simulink model "Electrical787"  (R2013a)
settings: Solver=ode45  StartTime=0.0  StopTime=MSSN.gen.time(end)  RelTol=1e-3
InitFcn:
  | load('SampleOutput.mat')
  | 
  | load('SampleFuelBurn.mat')
undefined symbols (not defined in the file): ailerons, B_737, elevator, FuelBurn, landing_gear, rudder, thrust_rev
libraries: PowerFlowLib x95, simulink x17
(part 17 of 17)

== system Electrical787/ELECTRICAL SYS /Engine Outputs ==
  Left_Wing_Toqrue_Nm : Inport
  Rght_Wing_Torque_Nm : Inport  Port=2
  APU_Torque_Nm : Inport  Port=3
  Bus Creator : BusCreator  Inputs=3
  Electrical : Outport
  wires:
  Rght_Wing_Torque_Nm/1 -> Bus Creator/2  "Right Wing Torq (Nm)"
  APU_Torque_Nm/1 -> Bus Creator/3  "APU Torq (Nm)"
  Left_Wing_Toqrue_Nm/1 -> Bus Creator/1  "Left Wing Torq (Nm)"
  Bus Creator/1 -> Electrical/1

== system Electrical787/ELECTRICAL SYS /Generation Unit P.M. ==
  engine speed : Inport
  idq0 : Inport  Port=2
  Temperature : Inport  Port=3
  Bus Creator : BusCreator  Inputs=3
  Bus Creator1 : BusCreator  Inputs=3
  Coeff of Resistance : Gain  Gain=3.85e-3
  Demux : Demux  Outputs=3
  Gain : Gain  Gain=200*2/3
  Gain1 : Gain  Gain=200
  Generator : Subsystem
      mask Display:
      | p = 0:0.1:(2*pi+0.1);
      | plot(sin(p), cos(p));
      | p1 = (-pi/8-0.1-0.2):0.1:(pi/8+0.1-0.2);
      | plot(0.8*sin(p1), 0.8*cos(p1), 0.8*sin(p1+pi), 0.8*cos(p1+pi));
      | p2 = sin((-pi/8-0.1-0.2+pi/8+0.1-0.2)/2);
      | p3 = sin((-pi/8-0.1-0.2+pi/8+0.1-0.2)/2+pi);
      | p4 = cos((-pi/8-0.1-0.2+pi/8+0.1-0.2)/2);
      | p5 = cos((-pi/8-0.1-0.2+pi/8+0.1-0.2)/2+pi);
      | plot(0.8*[p2, p3], 0.8*[p4, p5]);
      | port_label('output', 1, 'Vdq0');
      | port_label('output', 2, 'Te');
      | port_label('output', 3, 'Vfd');
      | port_label('output', 4, 'Ploss');
      | port_label('input', 1, 'idq0');
      | port_label('input', 2, 'w');
      | port_label('input', 3, 'ifd');
  Initial Temperature : Constant  Value=25
  Memory : Memory
  Permanent Magnet Synchronous Generator1 : PowerFlowLib/Energy & Power Systems/Electrical/Machines/Permanent Magnet Synchronous Generator1
  RPM_to_radps : Gain  Gain=pi/30
  Scope2 : Scope
      settings: TimeRange=100  YMin=0  YMax=5500  SaveName=ScopeData4
  Sum : Sum  Inputs=++|
  Sum1 : Sum
  Sum5 : Sum  Inputs=|+-
  Sum6 : Sum  Inputs=|++
  control1 : Constant
  data_sink : PowerFlowLib/Support Functions//Tools/data_sink
  one : Constant
  three-phase active rectifier Voltage Mode : PowerFlowLib/Energy & Power Systems/Electrical/Rectifiers/three-phase  active rectifier Voltage Mode  L=1  C=1e-4
  vdq0 : Outport
  engine torque : Outport  Port=2
  Ploss : Outport  Port=3
  wires:
  [R_temp_delta] -> Generator/4(Temp)
  Sum6/1 -> [R_temp_delta]
  one/1 -> Sum6/2
  Coeff of Resistance/1 -> Sum6/1
  Sum5/1 -> Coeff of Resistance/1
  Initial Temperature/1 -> Sum5/2
  Temperature/1 -> Sum5/1
  engine speed/1 -> RPM_to_radps/1
  Bus Creator1/1 -> Bus Creator/1  "vdq0 (V)"
  Demux/3 -> Bus Creator1/3  "v0"
  Demux/2 -> Bus Creator1/2  "vq"
  Demux/1 -> Bus Creator1/1  "vd"
  Bus Creator/1 -> data_sink/1
  Sum/1 -> engine torque/1
  RPM_to_radps/1 -> Scope2/1, Permanent Magnet Synchronous Generator1/2, Generator/2(w)
  Permanent Magnet Synchronous Generator1/1 -> three-phase active rectifier Voltage Mode/1
  control1/1 -> three-phase active rectifier Voltage Mode/2
  Generator/3(vfd') -> Gain1/1
  Gain1/1 -> three-phase active rectifier Voltage Mode/3
  Gain/1 -> Generator/3(ifd'), Bus Creator/3  "Excit current (A)"
  three-phase active rectifier Voltage Mode/1 -> Gain/1
  three-phase active rectifier Voltage Mode/2 -> Memory/1
  Permanent Magnet Synchronous Generator1/2 -> Sum/1
  Generator/2(Te) -> Sum/2
  idq0/1 -> Generator/1(idq0)
  Generator/1(vdq0) -> Demux/1, vdq0/1  "Vdq0 (V)"
  Permanent Magnet Synchronous Generator1/3 -> Sum1/1
  Generator/4(Ploss) -> Sum1/2
  Sum1/1 -> Bus Creator/2, Ploss/1  "Ploss (W)"
  Memory/1 -> Permanent Magnet Synchronous Generator1/1

== system Electrical787/ELECTRICAL SYS /Generation Unit P.M.1 ==
  engine speed : Inport
  idq0 : Inport  Port=2
  Temperature : Inport  Port=3
  Bus Creator : BusCreator  Inputs=3
  Bus Creator1 : BusCreator  Inputs=3
  Coeff of Resistance : Gain  Gain=3.85e-3
  Demux : Demux  Outputs=3
  Gain : Gain  Gain=200*2/3
  Gain1 : Gain  Gain=200
  Generator : Subsystem
      mask Display:
      | p = 0:0.1:(2*pi+0.1);
      | plot(sin(p), cos(p));
      | p1 = (-pi/8-0.1-0.2):0.1:(pi/8+0.1-0.2);
      | plot(0.8*sin(p1), 0.8*cos(p1), 0.8*sin(p1+pi), 0.8*cos(p1+pi));
      | p2 = sin((-pi/8-0.1-0.2+pi/8+0.1-0.2)/2);
      | p3 = sin((-pi/8-0.1-0.2+pi/8+0.1-0.2)/2+pi);
      | p4 = cos((-pi/8-0.1-0.2+pi/8+0.1-0.2)/2);
      | p5 = cos((-pi/8-0.1-0.2+pi/8+0.1-0.2)/2+pi);
      | plot(0.8*[p2, p3], 0.8*[p4, p5]);
      | port_label('output', 1, 'Vdq0');
      | port_label('output', 2, 'Te');
      | port_label('output', 3, 'Vfd');
      | port_label('output', 4, 'Ploss');
      | port_label('input', 1, 'idq0');
      | port_label('input', 2, 'w');
      | port_label('input', 3, 'ifd');
  Initial Temperature : Constant  Value=25
  Memory : Memory
  Permanent Magnet Synchronous Generator1 : PowerFlowLib/Energy & Power Systems/Electrical/Machines/Permanent Magnet Synchronous Generator1
  RPM_to_radps : Gain  Gain=pi/30
  Scope2 : Scope
      settings: TimeRange=100  YMin=0  YMax=5500  SaveName=ScopeData4
  Sum : Sum  Inputs=++|
  Sum1 : Sum
  Sum5 : Sum  Inputs=|+-
  Sum6 : Sum  Inputs=|++
  control1 : Constant
  data_sink : PowerFlowLib/Support Functions//Tools/data_sink
  one : Constant
  three-phase active rectifier Voltage Mode : PowerFlowLib/Energy & Power Systems/Electrical/Rectifiers/three-phase  active rectifier Voltage Mode  L=1  C=1e-4
  vdq0 : Outport
  engine torque : Outport  Port=2
  Ploss : Outport  Port=3
  wires:
  [R_temp_delta] -> Generator/4(Temp)
  Sum6/1 -> [R_temp_delta]
  one/1 -> Sum6/2
  Coeff of Resistance/1 -> Sum6/1
  Sum5/1 -> Coeff of Resistance/1
  Initial Temperature/1 -> Sum5/2
  Temperature/1 -> Sum5/1
  engine speed/1 -> RPM_to_radps/1
  Bus Creator1/1 -> Bus Creator/1  "vdq0 (V)"
  Demux/3 -> Bus Creator1/3  "v0"
  Demux/2 -> Bus Creator1/2  "vq"
  Demux/1 -> Bus Creator1/1  "vd"
  Bus Creator/1 -> data_sink/1
  Sum/1 -> engine torque/1
  RPM_to_radps/1 -> Scope2/1, Permanent Magnet Synchronous Generator1/2, Generator/2(w)
  Permanent Magnet Synchronous Generator1/1 -> three-phase active rectifier Voltage Mode/1
  control1/1 -> three-phase active rectifier Voltage Mode/2
  Generator/3(vfd') -> Gain1/1
  Gain1/1 -> three-phase active rectifier Voltage Mode/3
  Gain/1 -> Generator/3(ifd'), Bus Creator/3  "Excit current (A)"
  three-phase active rectifier Voltage Mode/1 -> Gain/1
  three-phase active rectifier Voltage Mode/2 -> Memory/1
  Permanent Magnet Synchronous Generator1/2 -> Sum/1
  Generator/2(Te) -> Sum/2
  idq0/1 -> Generator/1(idq0)
  Generator/1(vdq0) -> Demux/1, vdq0/1  "Vdq0 (V)"
  Permanent Magnet Synchronous Generator1/3 -> Sum1/1
  Generator/4(Ploss) -> Sum1/2
  Sum1/1 -> Bus Creator/2, Ploss/1  "Ploss (W)"
  Memory/1 -> Permanent Magnet Synchronous Generator1/1

== system Electrical787/ELECTRICAL SYS /Loads ==
  Constant{,1..3} (4 alike) : Constant  Value=[150 0 0]
  ElectricalSource1 : PowerFlowLib/Support Functions//Tools/ElectricalSource  Tag=Flow  Description=TwoPhase  load_loc=Cockpit  ACDC_load=DC
      link override From1: GotoTag=RightWing_ElecAC_9219
      link override From2: GotoTag=RightWing_ElecAC_5921
  ElectricalSource4 : PowerFlowLib/Support Functions//Tools/ElectricalSource  Tag=Flow  Description=TwoPhase  load_loc=RightWing  ACDC_load=AC
      link override From1: GotoTag=RightWing_ElecAC_9219
      link override From2: GotoTag=RightWing_ElecAC_5921
  ElectricalSource5 : PowerFlowLib/Support Functions//Tools/ElectricalSource  Tag=Flow  Description=TwoPhase  load_loc=RightWing  ACDC_load=AC
      link override From1: GotoTag=RightWing_ElecAC_9219
      link override From2: GotoTag=RightWing_ElecAC_5921
  ElectricalSource6 : PowerFlowLib/Support Functions//Tools/ElectricalSource  Tag=Flow  Description=TwoPhase  load_loc=Cabin  ACDC_load=DC
      link override From1: GotoTag=RightWing_ElecAC_9219
      link override From2: GotoTag=RightWing_ElecAC_5921
  Reactive Power : Gain  Gain=[0 1 0]
  Reactive Power1 : Gain  Gain=[0 1 0]
  "Real Power " : Gain  Gain=[0 1]
  "Real Power  " : Gain  Gain=[1 0 0]
  Real Power  1 : Gain  Gain=[1 0 0]
  Real Power 1 : Gain  Gain=[0 1]
  Sum : Sum  Inputs=|++
  Sum of Elements{,1..3} (4 alike) : Sum  Inputs=+
  Sum1 : Sum  Inputs=|++
  230 Vac Loads : Outport
  115 Vac Loads : Outport  Port=2
  270 Vdc Loads : Outport  Port=3
  28 Vdc Loads : Outport  Port=4
  wires:
  "Real Power  "/1 -> Sum/1
  Reactive Power/1 -> Sum/2
  Sum of Elements/1 -> "Real Power  "/1
  Sum of Elements1/1 -> Reactive Power/1
  Real Power  1/1 -> Sum1/1
  Reactive Power1/1 -> Sum1/2
  Sum of Elements2/1 -> Real Power  1/1
  Sum of Elements3/1 -> Reactive Power1/1
  ElectricalSource6/1 -> "Real Power "/1
  ElectricalSource4/2 -> Sum of Elements3/1
  ElectricalSource5/1 -> Sum of Elements/1
  ElectricalSource5/2 -> Sum of Elements1/1
  ElectricalSource4/1 -> Sum of Elements2/1
  ElectricalSource1/1 -> Real Power 1/1
  Constant/1 -> 230 Vac Loads/1
  Constant1/1 -> 115 Vac Loads/1
  Constant2/1 -> 270 Vdc Loads/1
  Constant3/1 -> 28 Vdc Loads/1

== system Electrical787/ELECTRICAL SYS /Thermal Interface ==
  Left_Wing_SCVGU_Ploss_W : Inport
  Right_Wing_SCVGU_Ploss_W : Inport  Port=2
  APU_Ploss_W : Inport  Port=3
  Inverter_Ploss_W : Inport  Port=4
  Battery1_Ploss_W : Inport  Port=5
  Battery2_Ploss_W : Inport  Port=6
  Backup_Battery_Ploss_W : Inport  Port=7
  Loadloss_W : Inport  Port=8
  Mux : Mux
  Sum : Sum
  Terminator{,1..3} (4 alike) : Terminator
  ThermalSink : PowerFlowLib/Support Functions//Tools/ThermalSink  Tag=Flow  Description=TwoPhase  load_loc=Cabin  units=Watts  unq_id=8332
  To Workspace : ToWorkspace  VariableName=Tot_Gen_Loss_W  SampleTime=10  SaveFormat=Structure With Time
  wires:
  Right_Wing_SCVGU_Ploss_W/1 -> Sum/2, Terminator1/1
  APU_Ploss_W/1 -> Terminator2/1
  Mux/1 -> ThermalSink/1
  Inverter_Ploss_W/1 -> Mux/1
  Battery1_Ploss_W/1 -> Mux/2
  Battery2_Ploss_W/1 -> Mux/3
  Backup_Battery_Ploss_W/1 -> Mux/4
  Loadloss_W/1 -> Terminator3/1
  Left_Wing_SCVGU_Ploss_W/1 -> Sum/1, Terminator/1
  Sum/1 -> To Workspace/1

== system Electrical787/Engine #1/Unit Conversion  ==
  Signal_in : Inport
  conv_fcn : Fcn  Expr=u(1)/745.69987
  Converted Signal Out : Outport
  wires:
  Signal_in/1 -> conv_fcn/1
  conv_fcn/1 -> Converted Signal Out/1

== system Electrical787/Engine #1/Unit Conversion 1 ==
  Signal_in : Inport
  conv_fcn : Fcn  Expr=u(1)/1.8
  Converted Signal Out : Outport
  wires:
  conv_fcn/1 -> Converted Signal Out/1
  Signal_in/1 -> conv_fcn/1

== system Electrical787/Engine #1/Unit Conversion 2 ==
  Signal_in : Inport
  conv_fcn : Fcn  Expr=u(1)/.45359237
  Converted Signal Out : Outport
  wires:
  conv_fcn/1 -> Converted Signal Out/1
  Signal_in/1 -> conv_fcn/1

== system Electrical787/Engine #1/Unit Conversion 3 ==
  Signal_in : Inport
  conv_fcn : Fcn  Expr=u(1)/.45359237
  Converted Signal Out : Outport
  wires:
  conv_fcn/1 -> Converted Signal Out/1
  Signal_in/1 -> conv_fcn/1

== system Electrical787/Engine #1/Unit Conversion 4 ==
  Signal_in : Inport
  conv_fcn : Fcn  Expr=u(1)/(1.450377e-1)
  Converted Signal Out : Outport
  wires:
  Signal_in/1 -> conv_fcn/1
  conv_fcn/1 -> Converted Signal Out/1

== system Electrical787/Engine #1/Unit Conversion 5 ==
  Signal_in : Inport
  conv_fcn : Fcn  Expr=u(1)*.45359237
  Converted Signal Out : Outport
  wires:
  Signal_in/1 -> conv_fcn/1
  conv_fcn/1 -> Converted Signal Out/1

== system Electrical787/Engine #2/Unit Conversion  ==
  Signal_in : Inport
  conv_fcn : Fcn  Expr=u(1)/745.69987
  Converted Signal Out : Outport
  wires:
  conv_fcn/1 -> Converted Signal Out/1
  Signal_in/1 -> conv_fcn/1

== system Electrical787/Engine #2/Unit Conversion 1 ==
  Signal_in : Inport
  conv_fcn : Fcn  Expr=u(1)/1.8
  Converted Signal Out : Outport
  wires:
  Signal_in/1 -> conv_fcn/1
  conv_fcn/1 -> Converted Signal Out/1

== system Electrical787/Engine #2/Unit Conversion 2 ==
  Signal_in : Inport
  conv_fcn : Fcn  Expr=u(1)/.45359237
  Converted Signal Out : Outport
  wires:
  Signal_in/1 -> conv_fcn/1
  conv_fcn/1 -> Converted Signal Out/1

== system Electrical787/Engine #2/Unit Conversion 3 ==
  Signal_in : Inport
  conv_fcn : Fcn  Expr=u(1)/.45359237
  Converted Signal Out : Outport
  wires:
  Signal_in/1 -> conv_fcn/1
  conv_fcn/1 -> Converted Signal Out/1

== system Electrical787/Engine #2/Unit Conversion 4 ==
  Signal_in : Inport
  conv_fcn : Fcn  Expr=u(1)/(1.450377e-1)
  Converted Signal Out : Outport
  wires:
  conv_fcn/1 -> Converted Signal Out/1
  Signal_in/1 -> conv_fcn/1

== system Electrical787/Engine #2/Unit Conversion 5 ==
  Signal_in : Inport
  conv_fcn : Fcn  Expr=u(1)*.45359237
  Converted Signal Out : Outport
  wires:
  conv_fcn/1 -> Converted Signal Out/1
  Signal_in/1 -> conv_fcn/1

== system Electrical787/ECS & FOS /Fuel Tanks//Pumps/FlowGenerator1 ==
  Bias : Bias  Bias=273.15
  Bus Creator1 : BusCreator
  Constant3 : Constant  Value=flowenthalpy
  Constant5 : Constant  Value=flowrate
  Constant6 : Constant  Value=flowtemp
  Constant7 : Constant  Value=flowpres
  FlowOut : Outport  Tag=Flow Out
  wires:
  Bias/1 -> Bus Creator1/2  "temp_K"
  Constant5/1 -> Bus Creator1/1  "mdot_kgps"
  Constant3/1 -> Bus Creator1/4  "H_kJpkg"
  Constant7/1 -> Bus Creator1/3  "pres_kPa"
  Constant6/1 -> Bias/1  "temp_C"
  Bus Creator1/1 -> FlowOut/1  "Outlet"

== system Electrical787/ECS & FOS /Fuel Tanks//Pumps/Fuel Control Left Wing ==
  FuelNeed : Inport
  FuelFromPump : Inport  Port=2
  Bus Creator : BusCreator  Inputs=3
  Bus Creator1 : BusCreator  Inputs=3
  Bus Selector : BusSelector  OutputSignals=mdot_kgps,temp_K,pres_kPa
  Gain : Gain
  Gain1 : Gain
  Saturation : Saturate  UpperLimit=inf  LowerLimit=0
  Sum : Sum  Inputs=|+-
  Switch : Switch  Criteria=u2 > Threshold
  Fuel2Engine : Outport
  Fuel2Tank : Outport  Port=2
  wires:
  Gain1/1 -> Bus Creator1/2  "temp_K"
  Gain/1 -> Bus Creator1/3  "pres_kPa"
  Bus Creator1/1 -> Fuel2Engine/1
  Bus Selector/3 -> Gain/1, Bus Creator/3  "<pres_kPa>"
  Switch/1 -> Bus Creator1/1  "mdot_kgps"
  Saturation/1 -> Bus Creator/1  "mdot_kgps"
  Bus Selector/2 -> Gain1/1, Bus Creator/2  "<temp_K>"
  Bus Creator/1 -> Fuel2Tank/1
  Sum/1 -> Switch/2, Saturation/1
  FuelNeed/1 -> Switch/1, Sum/2
  Bus Selector/1 -> Switch/3, Sum/1  "<mdot_kgps>"
  FuelFromPump/1 -> Bus Selector/1

== system Electrical787/ECS & FOS /Fuel Tanks//Pumps/Fuel Control Right Wing  ==
  FuelNeed : Inport
  FuelFromPump : Inport  Port=2
  Bus Creator : BusCreator  Inputs=3
  Bus Creator1 : BusCreator  Inputs=3
  Bus Selector : BusSelector  OutputSignals=mdot_kgps,temp_K,pres_kPa
  Gain : Gain
  Gain1 : Gain
  Saturation : Saturate  UpperLimit=inf  LowerLimit=0
  Sum : Sum  Inputs=|+-
  Switch : Switch  Criteria=u2 > Threshold
  Fuel2Engine : Outport
  Fuel2Tank : Outport  Port=2
  wires:
  FuelFromPump/1 -> Bus Selector/1
  Bus Selector/1 -> Sum/1, Switch/3  "<mdot_kgps>"
  FuelNeed/1 -> Sum/2, Switch/1
  Sum/1 -> Saturation/1, Switch/2
  Bus Creator/1 -> Fuel2Tank/1
  Bus Selector/2 -> Bus Creator/2, Gain1/1  "<temp_K>"
  Saturation/1 -> Bus Creator/1  "mdot_kgps"
  Switch/1 -> Bus Creator1/1  "mdot_kgps"
  Bus Selector/3 -> Bus Creator/3, Gain/1  "<pres_kPa>"
  Bus Creator1/1 -> Fuel2Engine/1
  Gain/1 -> Bus Creator1/3  "pres_kPa"
  Gain1/1 -> Bus Creator1/2  "temp_K"

== system Electrical787/ECS & FOS /Fuel Tanks//Pumps/Fuel Switch On//Off ==
  Right Wing Tank : Inport
  Center Tank : Inport  Port=2
  Left Wing Tank : Inport  Port=3
  Operating RPM : Constant  Value=6000
  Operating RPM1 : Constant  Value=6000
  Operating RPM2 : Constant  Value=6000
  Right Wing Fuel Pumps On/Off : Switch  Criteria=u2 ~= 0
  Right Wing Fuel Pumps On/Off1 : Switch  Criteria=u2 ~= 0
  Right Wing Fuel Pumps On/Off2 : Switch  Criteria=u2 ~= 0
  shut off : Constant  Value=0
  shut off1 : Constant  Value=0
  shut off2 : Constant  Value=0
  Right Wing RPM : Outport
  Left Wing RPM : Outport  Port=2
  Center RPM : Outport  Port=3
  wires:
  Operating RPM/1 -> Right Wing Fuel Pumps On/Off/1
  shut off/1 -> Right Wing Fuel Pumps On/Off/3
  Right Wing Tank/1 -> Right Wing Fuel Pumps On/Off/2
  Operating RPM1/1 -> Right Wing Fuel Pumps On/Off1/1
  shut off1/1 -> Right Wing Fuel Pumps On/Off1/3
  Center Tank/1 -> Right Wing Fuel Pumps On/Off1/2
  Operating RPM2/1 -> Right Wing Fuel Pumps On/Off2/1
  shut off2/1 -> Right Wing Fuel Pumps On/Off2/3
  Left Wing Tank/1 -> Right Wing Fuel Pumps On/Off2/2
  Right Wing Fuel Pumps On/Off/1 -> Right Wing RPM/1
  Right Wing Fuel Pumps On/Off1/1 -> Center RPM/1
  Right Wing Fuel Pumps On/Off2/1 -> Left Wing RPM/1

== system Electrical787/ECS & FOS /Fuel Tanks//Pumps/Pump Split ==
  Flow In : Inport
  Bus Creator : BusCreator  Inputs=3
  Bus Selector14 : BusSelector  OutputSignals=temp_K,mdot_kgps,pres_kPa
  Gain : Gain  Gain=0.5
  Flow Out : Outport
  wires:
  Bus Selector14/3 -> Bus Creator/3  "<pres_kPa>"
  Gain/1 -> Bus Creator/2  "mdot_kgps"
  Bus Selector14/1 -> Bus Creator/1  "<temp_K>"
  Bus Creator/1 -> Flow Out/1
  Bus Selector14/2 -> Gain/1  "<mdot_kgps>"
  Flow In/1 -> Bus Selector14/1

== system Electrical787/ECS & FOS /Fuel Tanks//Pumps/Pump Split1 ==
  Flow In : Inport
  Bus Creator : BusCreator  Inputs=3
  Bus Selector14 : BusSelector  OutputSignals=temp_K,mdot_kgps,pres_kPa
  Gain : Gain  Gain=0.5
  Flow Out : Outport
  wires:
  Flow In/1 -> Bus Selector14/1
  Bus Selector14/2 -> Gain/1  "<mdot_kgps>"
  Bus Creator/1 -> Flow Out/1
  Bus Selector14/1 -> Bus Creator/1  "<temp_K>"
  Gain/1 -> Bus Creator/2  "mdot_kgps"
  Bus Selector14/3 -> Bus Creator/3  "<pres_kPa>"

== system Electrical787/ECS & FOS /Fuel Tanks//Pumps/Pump Split2 ==
  Flow In : Inport
  Bus Creator : BusCreator  Inputs=3
  Bus Selector14 : BusSelector  OutputSignals=temp_K,mdot_kgps,pres_kPa
  Gain : Gain  Gain=0.5
  Flow Out : Outport
  wires:
  Bus Selector14/3 -> Bus Creator/3  "<pres_kPa>"
  Gain/1 -> Bus Creator/2  "mdot_kgps"
  Bus Selector14/1 -> Bus Creator/1  "<temp_K>"
  Bus Creator/1 -> Flow Out/1
  Bus Selector14/2 -> Gain/1  "<mdot_kgps>"
  Flow In/1 -> Bus Selector14/1

== system Electrical787/ECS & FOS /Left PACK/Distribution of bleed air ==
  Bleed to Valve : Inport
  Bleed to ACM : Inport  Port=2
  bleed_temp : Inport  Port=3
  bleed_pres : Inport  Port=4
  Bus Creator1 : BusCreator  Inputs=3
  Bus Creator2 : BusCreator  Inputs=3
  Scope : Scope  NumInputPorts=4
      settings: YMin=0~386.7~110~0.2  YMax=0.055~387.8~160~0.85  SaveName=ScopeData42  SampleInput=on  SampleTime=1
  Flow to Mix Junc. : Outport
  Flow to HX : Outport  Port=2
  wires:
  Bleed to ACM/1 -> Bus Creator2/1, Scope/4  "mdot_kgps"
  bleed_temp/1 -> Bus Creator2/2, Bus Creator1/2, Scope/2
  bleed_pres/1 -> Bus Creator2/3, Bus Creator1/3, Scope/3
  Bleed to Valve/1 -> Bus Creator1/1, Scope/1  "mdot_kgps"
  Bus Creator1/1 -> Flow to Mix Junc./1
  Bus Creator2/1 -> Flow to HX/1

== system Electrical787/ECS & FOS /Left PACK/Ram air inlet ==
  Temp_amb : Inport
  Temp_comp : Inport  Port=2
  2 : Constant  Value=T_35
  Bus Creator : BusCreator  Inputs=3
  Bus Selector4 : BusSelector  OutputSignals=temp_K
  Constant1 : Constant  Value=22.5
  Gain : Gain  Gain=0.95
  Gain1 : Gain
  Memory : Memory  X0=ram_air
  Subtract : Sum  Inputs=+-
  Switch : Switch  Criteria=u2 ~= 0  Threshold=30
  Flow Out : Outport
  wires:
  Temp_comp/1 -> Bus Selector4/1
  Bus Selector4/1 -> Subtract/1  "<temp_K>"
  2/1 -> Subtract/2
  Subtract/1 -> Switch/2
  Gain/1 -> Switch/3
  Switch/1 -> Memory/1
  Temp_amb/1 -> Bus Creator/1  "temp_K"
  Constant1/1 -> Bus Creator/2  "pres_kPa"
  Bus Creator/1 -> Flow Out/1
  Memory/1 -> Bus Creator/3, Gain1/1, Gain/1  "mdot_kgps"
  Gain1/1 -> Switch/1

== system Electrical787/ECS & FOS /Left PACK/Subsystem1 ==
  Bypass Ratio : Inport
  Air from PHX : Inport  Port=2
  Bus Creator : BusCreator  Inputs=3
  Bus Creator1 : BusCreator  Inputs=3
  Bus Selector : BusSelector  OutputSignals=mdot_kgps,temp_K,pres_kPa
  Fcn1 : Fcn  Expr=1-u(1)
  Gain : Gain
  Gain1 : Gain
  Gain2 : Gain
  Product : Product  RndMeth=Zero
  Product1 : Product  RndMeth=Zero
  Saturation : Saturate  UpperLimit=inf  LowerLimit=eps
  Air to Mix Junc : Outport
  Air to Comp : Outport  Port=2
  wires:
  Gain1/1 -> Bus Creator1/2  "temp_K"
  Gain/1 -> Bus Creator1/3  "pres_kPa"
  Bus Creator1/1 -> Air to Mix Junc/1
  Bus Selector/3 -> Gain/1, Gain2/1  "<pres_kPa>"
  Product1/1 -> Bus Creator1/1  "mdot_kgps"
  Saturation/1 -> Bus Creator/1  "mdot_kgps"
  Bus Selector/2 -> Gain1/1, Bus Creator/2  "<temp_K>"
  Bus Creator/1 -> Air to Comp/1
  Bus Selector/1 -> Product/2, Product1/1  "<mdot_kgps>"
  Air from PHX/1 -> Bus Selector/1
  Product/1 -> Saturation/1
  Bypass Ratio/1 -> Fcn1/1, Product1/2
  Fcn1/1 -> Product/1
  Gain2/1 -> Bus Creator/3  "pres_kPa"

== system Electrical787/ECS & FOS /Left PACK/User-set_ supply_pressure ==
  Flow In : Inport
  Cabin Pres. : Inport  Port=2
  Bus Creator4 : BusCreator  Inputs=3
  Bus Selector3 : BusSelector  OutputSignals=mdot_kgps,temp_K
  Gain1 : Gain  Gain=1.1
  Flow Out : Outport
  wires:
  Bus Selector3/1 -> Bus Creator4/1  "<mdot_kgps>"
  Bus Selector3/2 -> Bus Creator4/2  "<temp_K>"
  Gain1/1 -> Bus Creator4/3  "pres_kPa"
  Flow In/1 -> Bus Selector3/1
  Bus Creator4/1 -> Flow Out/1
  Cabin Pres./1 -> Gain1/1

== system Electrical787/ECS & FOS /Left PACK/Valve1 ==
  Flow In : Inport
  Bus Creator2 : BusCreator  Inputs=3
  Bus Selector2 : BusSelector  OutputSignals=mdot_kgps,pres_kPa,temp_K
  Math Functin : Math  Operator=pow  SaturateOnIntegerOverflow=on
  Product : Product  RndMeth=Zero
  Sum : Sum  Inputs=|-+
  "Value?? -- MAW" : Constant  Value=50
  get u : Gain
  mass_flow_rate1 : Constant  Value=2
  Flow Out : Outport
  wires:
  Bus Creator2/1 -> Flow Out/1
  Flow In/1 -> Bus Selector2/1
  Bus Selector2/1 -> Bus Creator2/1, get u/1  "<mdot_kgps>"
  get u/1 -> Math Functin/1
  mass_flow_rate1/1 -> Math Functin/2
  Math Functin/1 -> Product/2
  Product/1 -> Sum/1
  Bus Selector2/2 -> Sum/2  "<pres_kPa>"
  Sum/1 -> Bus Creator2/2  "pres_kPa"
  Bus Selector2/3 -> Bus Creator2/3  "<temp_K>"
  "Value?? -- MAW"/1 -> Product/1

== system Electrical787/ECS & FOS /Right PACK/Distribution of bleed air ==
  Bleed to Valve : Inport
  Bleed to ACM : Inport  Port=2
  bleed_temp : Inport  Port=3
  bleed_pres : Inport  Port=4
  Bus Creator1 : BusCreator  Inputs=3
  Bus Creator2 : BusCreator  Inputs=3
  Scope : Scope  NumInputPorts=4
      settings: YMin=0~386.7~110~0.2  YMax=0.055~387.8~160~0.85  SaveName=ScopeData42  SampleInput=on  SampleTime=1
  Flow to Mix Junc. : Outport
  Flow to HX : Outport  Port=2
  wires:
  Bus Creator2/1 -> Flow to HX/1
  Bus Creator1/1 -> Flow to Mix Junc./1
  Bleed to Valve/1 -> Scope/1, Bus Creator1/1  "mdot_kgps"
  bleed_pres/1 -> Scope/3, Bus Creator1/3, Bus Creator2/3
  bleed_temp/1 -> Scope/2, Bus Creator1/2, Bus Creator2/2
  Bleed to ACM/1 -> Scope/4, Bus Creator2/1  "mdot_kgps"

== system Electrical787/ECS & FOS /Right PACK/Ram air inlet ==
  Temp_amb : Inport
  Temp_comp : Inport  Port=2
  2 : Constant  Value=T_35
  Bus Creator : BusCreator  Inputs=3
  Bus Selector4 : BusSelector  OutputSignals=temp_K
  Constant1 : Constant  Value=22.5
  Gain : Gain  Gain=0.95
  Gain1 : Gain
  Memory : Memory  X0=ram_air
  Subtract : Sum  Inputs=+-
  Switch : Switch  Criteria=u2 ~= 0  Threshold=30
  Flow Out : Outport
  wires:
  Gain1/1 -> Switch/1
  Memory/1 -> Gain/1, Gain1/1, Bus Creator/3  "mdot_kgps"
  Bus Creator/1 -> Flow Out/1
  Constant1/1 -> Bus Creator/2  "pres_kPa"
  Temp_amb/1 -> Bus Creator/1  "temp_K"
  Switch/1 -> Memory/1
  Gain/1 -> Switch/3
  Subtract/1 -> Switch/2
  2/1 -> Subtract/2
  Bus Selector4/1 -> Subtract/1  "<temp_K>"
  Temp_comp/1 -> Bus Selector4/1

== system Electrical787/ECS & FOS /Right PACK/Subsystem1 ==
  Bypass Ratio : Inport
  Air from PHX : Inport  Port=2
  Bus Creator : BusCreator  Inputs=3
  Bus Creator1 : BusCreator  Inputs=3
  Bus Selector : BusSelector  OutputSignals=mdot_kgps,temp_K,pres_kPa
  Fcn1 : Fcn  Expr=1-u(1)
  Gain : Gain
  Gain1 : Gain
  Gain2 : Gain
  Product : Product  RndMeth=Zero
  Product1 : Product  RndMeth=Zero
  Saturation : Saturate  UpperLimit=inf  LowerLimit=eps
  Air to Mix Junc : Outport
  Air to Comp : Outport  Port=2
  wires:
  Gain2/1 -> Bus Creator/3  "pres_kPa"
  Fcn1/1 -> Product/1
  Bypass Ratio/1 -> Product1/2, Fcn1/1
  Product/1 -> Saturation/1
  Air from PHX/1 -> Bus Selector/1
  Bus Selector/1 -> Product1/1, Product/2  "<mdot_kgps>"
  Bus Creator/1 -> Air to Comp/1
  Bus Selector/2 -> Bus Creator/2, Gain1/1  "<temp_K>"
  Saturation/1 -> Bus Creator/1  "mdot_kgps"
  Product1/1 -> Bus Creator1/1  "mdot_kgps"
  Bus Selector/3 -> Gain2/1, Gain/1  "<pres_kPa>"
  Bus Creator1/1 -> Air to Mix Junc/1
  Gain/1 -> Bus Creator1/3  "pres_kPa"
  Gain1/1 -> Bus Creator1/2  "temp_K"

== system Electrical787/ECS & FOS /Right PACK/User-set_ supply_pressure ==
  Flow In : Inport
  Cabin Pres. : Inport  Port=2
  Bus Creator4 : BusCreator  Inputs=3
  Bus Selector3 : BusSelector  OutputSignals=mdot_kgps,temp_K
  Gain1 : Gain  Gain=1.1
  Flow Out : Outport
  wires:
  Cabin Pres./1 -> Gain1/1
  Bus Creator4/1 -> Flow Out/1
  Flow In/1 -> Bus Selector3/1
  Gain1/1 -> Bus Creator4/3  "pres_kPa"
  Bus Selector3/2 -> Bus Creator4/2  "<temp_K>"
  Bus Selector3/1 -> Bus Creator4/1  "<mdot_kgps>"

== system Electrical787/ECS & FOS /Right PACK/Valve1 ==
  Flow In : Inport
  Bus Creator2 : BusCreator  Inputs=3
  Bus Selector2 : BusSelector  OutputSignals=mdot_kgps,pres_kPa,temp_K
  Math Functin : Math  Operator=pow  SaturateOnIntegerOverflow=on
  Product : Product  RndMeth=Zero
  Sum : Sum  Inputs=|-+
  "Value?? -- MAW" : Constant  Value=50
  get u : Gain
  mass_flow_rate1 : Constant  Value=2
  Flow Out : Outport
  wires:
  "Value?? -- MAW"/1 -> Product/1
  Bus Selector2/3 -> Bus Creator2/3  "<temp_K>"
  Sum/1 -> Bus Creator2/2  "pres_kPa"
  Bus Selector2/2 -> Sum/2  "<pres_kPa>"
  Product/1 -> Sum/1
  Math Functin/1 -> Product/2
  mass_flow_rate1/1 -> Math Functin/2
  get u/1 -> Math Functin/1
  Bus Selector2/1 -> get u/1, Bus Creator2/1  "<mdot_kgps>"
  Flow In/1 -> Bus Selector2/1
  Bus Creator2/1 -> Flow Out/1

== system Electrical787/ECS & FOS /Thermal_sources_from Electrical_power_model1/ThermalSource ==
  LoadBus : BusCreator  Inputs=1
  Load : Outport
  wires:
  LoadBus/1 -> Load/1

== system Electrical787/ECS & FOS /Thermal_sources_from Electrical_power_model1/ThermalSource3 ==
  LoadBus : BusCreator  Inputs=1
  Load : Outport
  wires:
  LoadBus/1 -> Load/1

== system Electrical787/ECS & FOS /Thermal_sources_from Electrical_power_model1/ThermalSource4 ==
  LoadBus : BusCreator  Inputs=1
  Load : Outport
  wires:
  LoadBus/1 -> Load/1

== system Electrical787/ECS & FOS /Thermal_sources_from Electrical_power_model1/ThermalSource5 ==
  LoadBus : BusCreator  Inputs=1
  Load : Outport
  wires:
  LoadBus/1 -> Load/1

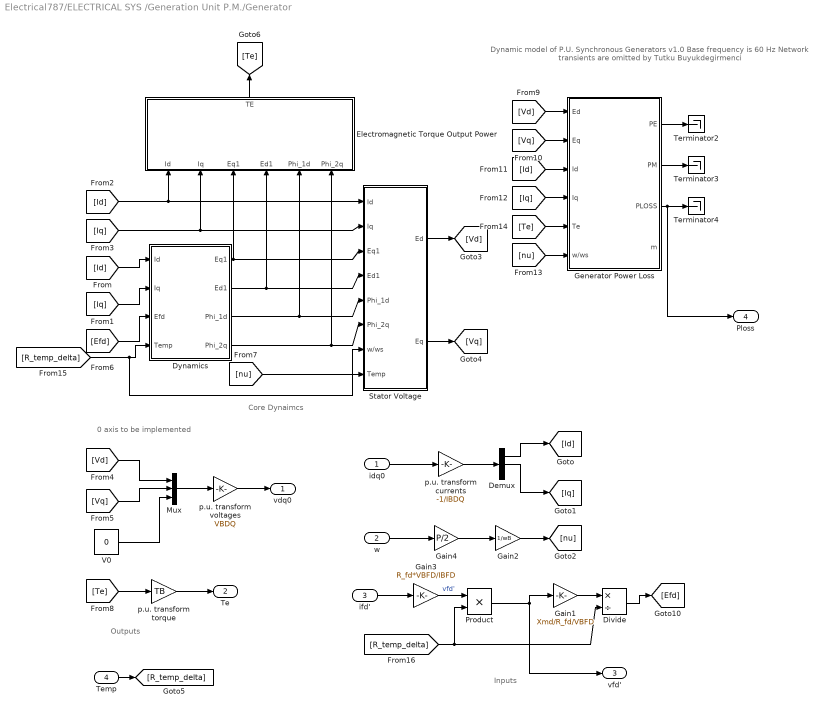
== system Electrical787/ELECTRICAL SYS /Generation Unit P.M./Generator ==
  note: 0 axis to be implemented
  note: Inputs
  note: Outputs
  note: Core Dynaimcs
  note: Dynamic model of P.U. Synchronous Generators v1.0
      | Base frequency is 60 Hz
      | Network transients are omitted
      | by Tutku Buyukdegirmenci
  idq0 : Inport
  w : Inport  Port=2
  ifd' : Inport  Port=3
  Temp : Inport  Port=4
  Demux : Demux  Outputs=3
  Divide : Product  Inputs=*/
  Dynamics : Subsystem
  Electromagnetic Torque Output Power : Subsystem
  Gain1 : Gain  Gain=Xmd/R_fd/VBFD
  Gain2 : Gain  Gain=1/wB
  Gain3 : Gain  Gain=R_fd*VBFD/IBFD
  Gain4 : Gain  Gain=P/2
  Generator Power Loss : Subsystem
  Mux : Mux  Inputs=3
  Product : Product
  Stator Voltage : Subsystem
  Terminator2 : Terminator
  Terminator3 : Terminator
  Terminator4 : Terminator
  V0 : Constant  Value=0
  p.u. transform currents : Gain  Gain=-1/IBDQ
  p.u. transform torque : Gain  Gain=TB
  p.u. transform voltages : Gain  Gain=VBDQ
  vdq0 : Outport
  Te : Outport  Port=2
  vfd' : Outport  Port=3
  Ploss : Outport  Port=4
  wires:
  [R_temp_delta] -> Dynamics/4(Temp), Stator Voltage/8(Temp)
  [R_temp_delta] -> Product/2, Divide/2
  Product/1 -> vfd'/1, Gain1/1
  Gain3/1 -> Product/1  "vfd'"
  Divide/1 -> [Efd]
  Gain1/1 -> Divide/1
  Temp/1 -> [R_temp_delta]
  Dynamics/1(Eq1) -> Stator Voltage/3(Eq1), Electromagnetic Torque Output Power/3(Eq1)
  Dynamics/2(Ed1) -> Stator Voltage/4(Ed1), Electromagnetic Torque Output Power/4(Ed1)
  Dynamics/3(Phi_1d) -> Stator Voltage/5(Phi_1d), Electromagnetic Torque Output Power/5(Phi_1d)
  Dynamics/4(Phi_2q) -> Stator Voltage/6(Phi_2q), Electromagnetic Torque Output Power/6(Phi_2q)
  Stator Voltage/2(Eq) -> [Vq]
  Stator Voltage/1(Ed) -> [Vd]
  w/1 -> Gain4/1
  Demux/1 -> [Id]
  Demux/2 -> [Iq]
  Gain2/1 -> [nu]
  [Id] -> Dynamics/1(Id)
  [Iq] -> Dynamics/2(Iq)
  [Id] -> Stator Voltage/1(Id), Electromagnetic Torque Output Power/1(Id)
  [Iq] -> Stator Voltage/2(Iq), Electromagnetic Torque Output Power/2(Iq)
  Mux/1 -> p.u. transform voltages/1
  [Vd] -> Mux/1
  [Vq] -> Mux/2
  V0/1 -> Mux/3
  [nu] -> Stator Voltage/7(w/ws)
  Electromagnetic Torque Output Power/1(TE) -> [Te]
  [Te] -> p.u. transform torque/1
  p.u. transform currents/1 -> Demux/1
  p.u. transform torque/1 -> Te/1
  [Vd] -> Generator Power Loss/1(Ed)
  [Vq] -> Generator Power Loss/2(Eq)
  [Id] -> Generator Power Loss/3(Id)
  [Iq] -> Generator Power Loss/4(Iq)
  [nu] -> Generator Power Loss/6(w/ws)
  [Te] -> Generator Power Loss/5(Te)
  Generator Power Loss/1(PE) -> Terminator2/1
  Generator Power Loss/2(PM) -> Terminator3/1
  Generator Power Loss/3(PLOSS) -> Terminator4/1, Ploss/1
  p.u. transform voltages/1 -> vdq0/1
  idq0/1 -> p.u. transform currents/1
  ifd'/1 -> Gain3/1
  [Efd] -> Dynamics/3(Efd)
  Gain4/1 -> Gain2/1

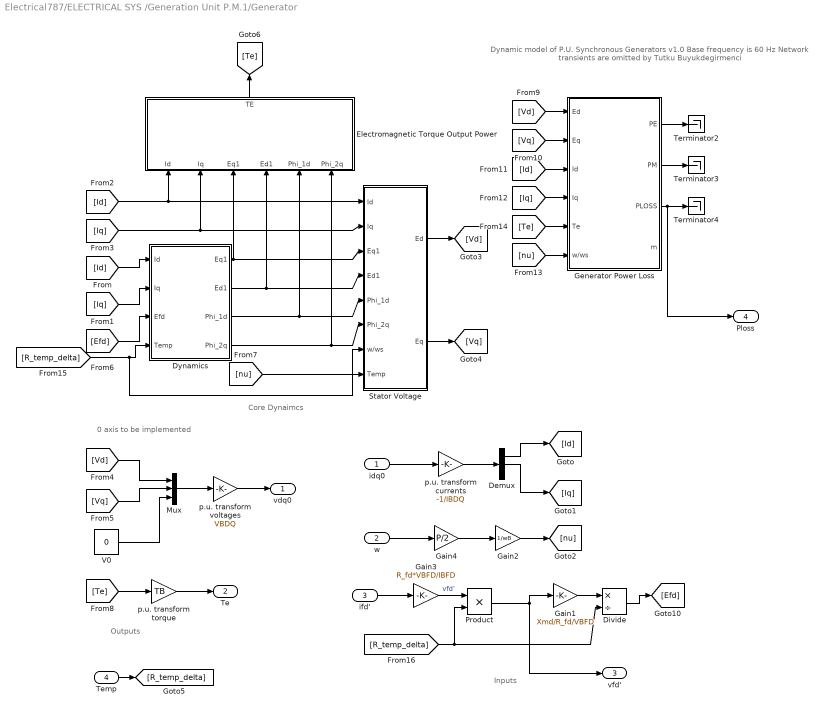
== system Electrical787/ELECTRICAL SYS /Generation Unit P.M.1/Generator ==
  note: 0 axis to be implemented
  note: Inputs
  note: Outputs
  note: Core Dynaimcs
  note: Dynamic model of P.U. Synchronous Generators v1.0
      | Base frequency is 60 Hz
      | Network transients are omitted
      | by Tutku Buyukdegirmenci
  idq0 : Inport
  w : Inport  Port=2
  ifd' : Inport  Port=3
  Temp : Inport  Port=4
  Demux : Demux  Outputs=3
  Divide : Product  Inputs=*/
  Dynamics : Subsystem
  Electromagnetic Torque Output Power : Subsystem
  Gain1 : Gain  Gain=Xmd/R_fd/VBFD
  Gain2 : Gain  Gain=1/wB
  Gain3 : Gain  Gain=R_fd*VBFD/IBFD
  Gain4 : Gain  Gain=P/2
  Generator Power Loss : Subsystem
  Mux : Mux  Inputs=3
  Product : Product
  Stator Voltage : Subsystem
  Terminator2 : Terminator
  Terminator3 : Terminator
  Terminator4 : Terminator
  V0 : Constant  Value=0
  p.u. transform currents : Gain  Gain=-1/IBDQ
  p.u. transform torque : Gain  Gain=TB
  p.u. transform voltages : Gain  Gain=VBDQ
  vdq0 : Outport
  Te : Outport  Port=2
  vfd' : Outport  Port=3
  Ploss : Outport  Port=4
  wires:
  [R_temp_delta] -> Dynamics/4(Temp), Stator Voltage/8(Temp)
  [R_temp_delta] -> Product/2, Divide/2
  Product/1 -> vfd'/1, Gain1/1
  Gain3/1 -> Product/1  "vfd'"
  Divide/1 -> [Efd]
  Gain1/1 -> Divide/1
  Temp/1 -> [R_temp_delta]
  Dynamics/1(Eq1) -> Stator Voltage/3(Eq1), Electromagnetic Torque Output Power/3(Eq1)
  Dynamics/2(Ed1) -> Stator Voltage/4(Ed1), Electromagnetic Torque Output Power/4(Ed1)
  Dynamics/3(Phi_1d) -> Stator Voltage/5(Phi_1d), Electromagnetic Torque Output Power/5(Phi_1d)
  Dynamics/4(Phi_2q) -> Stator Voltage/6(Phi_2q), Electromagnetic Torque Output Power/6(Phi_2q)
  Stator Voltage/2(Eq) -> [Vq]
  Stator Voltage/1(Ed) -> [Vd]
  w/1 -> Gain4/1
  Demux/1 -> [Id]
  Demux/2 -> [Iq]
  Gain2/1 -> [nu]
  [Id] -> Dynamics/1(Id)
  [Iq] -> Dynamics/2(Iq)
  [Id] -> Stator Voltage/1(Id), Electromagnetic Torque Output Power/1(Id)
  [Iq] -> Stator Voltage/2(Iq), Electromagnetic Torque Output Power/2(Iq)
  Mux/1 -> p.u. transform voltages/1
  [Vd] -> Mux/1
  [Vq] -> Mux/2
  V0/1 -> Mux/3
  [nu] -> Stator Voltage/7(w/ws)
  Electromagnetic Torque Output Power/1(TE) -> [Te]
  [Te] -> p.u. transform torque/1
  p.u. transform currents/1 -> Demux/1
  p.u. transform torque/1 -> Te/1
  [Vd] -> Generator Power Loss/1(Ed)
  [Vq] -> Generator Power Loss/2(Eq)
  [Id] -> Generator Power Loss/3(Id)
  [Iq] -> Generator Power Loss/4(Iq)
  [nu] -> Generator Power Loss/6(w/ws)
  [Te] -> Generator Power Loss/5(Te)
  Generator Power Loss/1(PE) -> Terminator2/1
  Generator Power Loss/2(PM) -> Terminator3/1
  Generator Power Loss/3(PLOSS) -> Terminator4/1, Ploss/1
  p.u. transform voltages/1 -> vdq0/1
  idq0/1 -> p.u. transform currents/1
  ifd'/1 -> Gain3/1
  [Efd] -> Dynamics/3(Efd)
  Gain4/1 -> Gain2/1

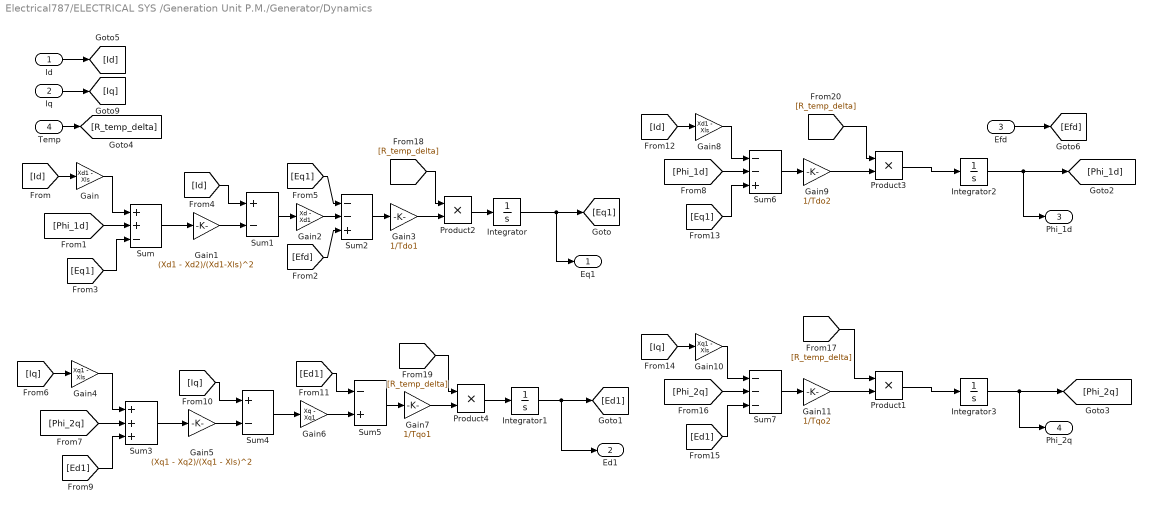
== system Electrical787/ELECTRICAL SYS /Generation Unit P.M./Generator/Dynamics ==
  Id : Inport
  Iq : Inport  Port=2
  Efd : Inport  Port=3
  Temp : Inport  Port=4
  Gain : Gain  Gain=Xd1 - Xls
  Gain1 : Gain  Gain=(Xd1 - Xd2)/(Xd1-Xls)^2
  Gain10 : Gain  Gain=Xq1 - Xls
  Gain11 : Gain  Gain=1/Tqo2
  Gain2 : Gain  Gain=Xd - Xd1
  Gain3 : Gain  Gain=1/Tdo1
  Gain4 : Gain  Gain=Xq1 - Xls
  Gain5 : Gain  Gain=(Xq1 - Xq2)/(Xq1 - Xls)^2
  Gain6 : Gain  Gain=Xq - Xq1
  Gain7 : Gain  Gain=1/Tqo1
  Gain8 : Gain  Gain=Xd1 - Xls
  Gain9 : Gain  Gain=1/Tdo2
  Integrator{,1..3} (4 alike) : Integrator
  Product{1..4} (4 alike) : Product
  Sum : Sum  Inputs=++-
  Sum1 : Sum  Inputs=+-
  Sum2 : Sum  Inputs=--+
  Sum3 : Sum  Inputs=+++
  Sum4 : Sum  Inputs=+-
  Sum5 : Sum  Inputs=-+
  Sum6 : Sum  Inputs=--+
  Sum7 : Sum  Inputs=---
  Eq1 : Outport
  Ed1 : Outport  Port=2
  Phi_1d : Outport  Port=3
  Phi_2q : Outport  Port=4
  wires:
  Product4/1 -> Integrator1/1
  Gain7/1 -> Product4/2
  [R_temp_delta] -> Product4/1
  Product2/1 -> Integrator/1
  Gain3/1 -> Product2/2
  [R_temp_delta] -> Product2/1
  Product1/1 -> Integrator3/1
  Gain11/1 -> Product1/2
  [R_temp_delta] -> Product1/1
  Product3/1 -> Integrator2/1
  Gain9/1 -> Product3/2
  [R_temp_delta] -> Product3/1
  Temp/1 -> [R_temp_delta]
  [Phi_1d] -> Sum/2
  Gain/1 -> Sum/1
  Integrator/1 -> Eq1/1, [Eq1]
  [Id] -> Gain/1
  [Eq1] -> Sum/3
  Sum/1 -> Gain1/1
  [Id] -> Sum1/1
  Gain1/1 -> Sum1/2
  Sum1/1 -> Gain2/1
  [Eq1] -> Sum2/1
  Gain2/1 -> Sum2/2
  [Efd] -> Sum2/3
  Sum2/1 -> Gain3/1
  Integrator1/1 -> Ed1/1, [Ed1]
  [Iq] -> Gain4/1
  Gain4/1 -> Sum3/1
  [Phi_2q] -> Sum3/2
  [Ed1] -> Sum3/3
  Sum3/1 -> Gain5/1
  [Iq] -> Sum4/1
  Gain5/1 -> Sum4/2
  Sum4/1 -> Gain6/1
  [Ed1] -> Sum5/1
  Gain6/1 -> Sum5/2
  Sum5/1 -> Gain7/1
  [Id] -> Gain8/1
  Gain8/1 -> Sum6/1
  [Phi_1d] -> Sum6/2
  [Eq1] -> Sum6/3
  Sum6/1 -> Gain9/1
  Integrator2/1 -> [Phi_1d], Phi_1d/1
  [Iq] -> Gain10/1
  Gain10/1 -> Sum7/1
  [Phi_2q] -> Sum7/2
  [Ed1] -> Sum7/3
  Sum7/1 -> Gain11/1
  Integrator3/1 -> [Phi_2q], Phi_2q/1
  Id/1 -> [Id]
  Iq/1 -> [Iq]
  Efd/1 -> [Efd]

== system Electrical787/ELECTRICAL SYS /Generation Unit P.M./Generator/Electromagnetic Torque Output Power ==
  note: Torque from Field Winding
  note: Torque from Damper Windings
  Id : Inport
  Iq : Inport  Port=2
  Eq1 : Inport  Port=3
  Ed1 : Inport  Port=4
  Phi_1d : Inport  Port=5
  Phi_2q : Inport  Port=6
  Gain : Gain  Gain=(Xd2 - Xls)/(Xd1 - Xls)
  Gain1 : Gain  Gain=(Xq2 - Xls)/(Xq1 - Xls)
  Gain2 : Gain  Gain=(Xd1 - Xd2)/(Xd1-Xls)
  Gain3 : Gain  Gain=(Xq1 - Xq2)/(Xq1-Xls)
  Gain4 : Gain  Gain=(Xq2 - Xd2)
  Product{,1..4} (5 alike) : Product  RndMeth=Zero
  Sum : Sum
  Sum1 : Sum  Inputs=+-+
  Sum2 : Sum
  TE : Outport
  wires:
  Id/1 -> [Id]
  Eq1/1 -> [Eq1]
  Ed1/1 -> [Ed1]
  Phi_1d/1 -> [Phi_1d]
  Phi_2q/1 -> [Phi_2q]
  Iq/1 -> [Iq]
  [Eq1] -> Product/1
  [Iq] -> Product/2
  Product/1 -> Gain/1
  [Ed1] -> Product1/1
  [Id] -> Product1/2
  Product1/1 -> Gain1/1
  [Iq] -> Product2/1
  [Phi_1d] -> Product2/2
  Product2/1 -> Gain2/1
  [Id] -> Product3/1
  [Phi_2q] -> Product3/2
  Product3/1 -> Gain3/1
  [Id] -> Product4/1
  [Iq] -> Product4/2
  Product4/1 -> Gain4/1
  Gain3/1 -> Sum1/2
  Gain2/1 -> Sum1/1
  Gain4/1 -> Sum1/3
  Gain/1 -> Sum/1
  Gain1/1 -> Sum/2
  Sum/1 -> Sum2/1
  Sum1/1 -> Sum2/2
  Sum2/1 -> TE/1

== system Electrical787/ELECTRICAL SYS /Generation Unit P.M./Generator/Generator Power Loss ==
  Ed : Inport
  Eq : Inport  Port=2
  Id : Inport  Port=3
  Iq : Inport  Port=4
  Te : Inport  Port=5
  w/ws : Inport  Port=6
  Bus Creator : BusCreator  Inputs=6
  Gain1 : Gain  Gain=SB
  Gain2 : Gain  Gain=SB
  Gain3 : Gain  Gain=SB
  Product : Product  RndMeth=Zero
  Product1 : Product  RndMeth=Zero
  Product2 : Product  RndMeth=Zero
  Sum1 : Sum  Inputs=-+
  Sum2 : Sum
  PE : Outport
  PM : Outport  Port=2
  PLOSS : Outport  Port=3
  m : Outport  Port=4
  wires:
  Ed/1 -> [Ed]
  Eq/1 -> [Eq]
  Id/1 -> [Id]
  Iq/1 -> [Iq]
  Te/1 -> [Te]
  w/ws/1 -> [nu]
  [Ed] -> Product/1
  [Id] -> Product/2
  [Eq] -> Product1/1
  [Iq] -> Product1/2
  [Te] -> Product2/1
  [nu] -> Product2/2
  Product/1 -> Sum2/1
  Product1/1 -> Sum2/2
  Sum2/1 -> Sum1/1, Gain1/1
  Product2/1 -> Sum1/2, Gain3/1
  Sum1/1 -> Gain2/1
  [Ed] -> Bus Creator/1  "Vd"
  [Id] -> Bus Creator/2  "Id"
  [Eq] -> Bus Creator/3  "Vq"
  [Iq] -> Bus Creator/4  "Iq"
  [Te] -> Bus Creator/5  "Te"
  [nu] -> Bus Creator/6  "nu"
  Bus Creator/1 -> m/1
  Gain2/1 -> PLOSS/1
  Gain1/1 -> PE/1
  Gain3/1 -> PM/1

== system Electrical787/ELECTRICAL SYS /Generation Unit P.M./Generator/Stator Voltage ==
  Id : Inport
  Iq : Inport  Port=2
  Eq1 : Inport  Port=3
  Ed1 : Inport  Port=4
  Phi_1d : Inport  Port=5
  Phi_2q : Inport  Port=6
  w/ws : Inport  Port=7
  Temp : Inport  Port=8
  Gain : Gain  Gain=(Xq2 - Xls)/(Xq1 - Xls)
  Gain1 : Gain  Gain=(Xq1 - Xq2)/(Xq1 - Xls)
  Gain2 : Gain  Gain=(Xq2 - Xd2)
  Gain3 : Gain  Gain=(Xd2 - Xls)/(Xd1 - Xls)
  Gain4 : Gain  Gain=(Xd1 - Xd2)/(Xd1 - Xls)
  Gain5 : Gain  Gain=Rs
  Gain6 : Gain  Gain=Xd2
  Gain7 : Gain  Gain=Rs
  Gain8 : Gain  Gain=Xd2
  Product{,1..3,5} (5 alike) : Product  RndMeth=Zero
  Product4 : Product
  Sum : Sum
  Sum1 : Sum  Inputs=+-+
  Sum2 : Sum  Inputs=--+
  Sum3 : Sum  Inputs=-++
  Ed : Outport
  Eq : Outport  Port=2
  wires:
  Iq/1 -> Gain6/1, Product5/2, Gain2/1
  Product5/1 -> Gain7/1
  Product4/1 -> Sum3/1
  Gain5/1 -> Product4/1
  Temp/1 -> Product4/2, Product5/1
  Gain2/1 -> Sum1/3
  Ed1/1 -> Gain/1
  Phi_2q/1 -> Gain1/1
  Eq1/1 -> Gain3/1
  Phi_1d/1 -> Gain4/1
  Gain4/1 -> Sum/2
  Gain3/1 -> Sum/1
  Gain/1 -> Sum1/1
  Gain1/1 -> Sum1/2
  Sum/1 -> Product/1
  Sum1/1 -> Product1/1
  w/ws/1 -> Product1/2, Product/2, Product3/2, Product2/1
  Product/1 -> Sum2/3
  Id/1 -> Gain5/1, Gain8/1
  Gain6/1 -> Product2/2
  Gain8/1 -> Product3/1
  Product1/1 -> Sum3/2
  Product2/1 -> Sum3/3
  Sum3/1 -> Ed/1  "Vd"
  Sum2/1 -> Eq/1  "Vq"
  Product3/1 -> Sum2/1
  Gain7/1 -> Sum2/2

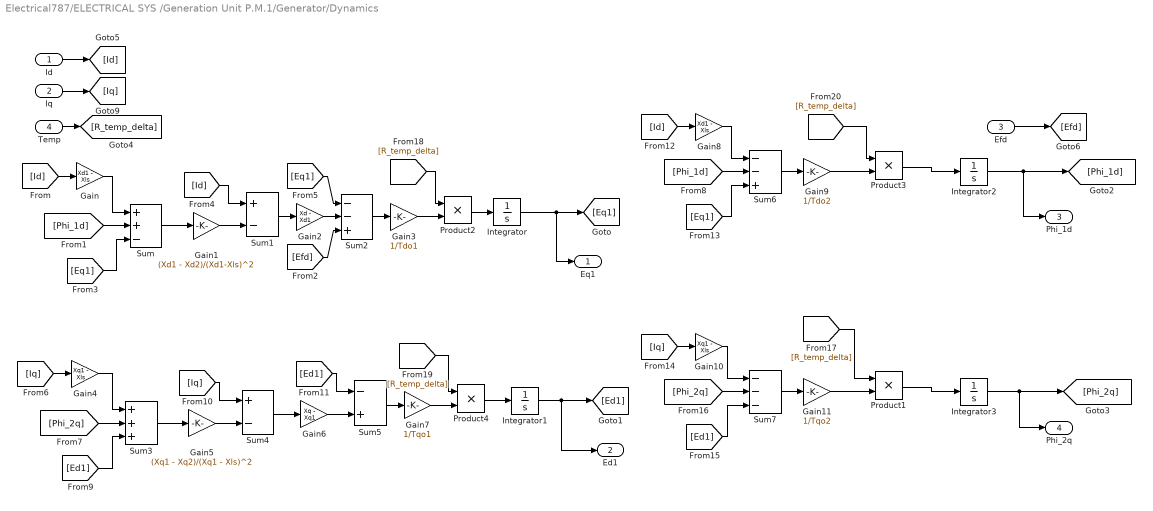
== system Electrical787/ELECTRICAL SYS /Generation Unit P.M.1/Generator/Dynamics ==
  Id : Inport
  Iq : Inport  Port=2
  Efd : Inport  Port=3
  Temp : Inport  Port=4
  Gain : Gain  Gain=Xd1 - Xls
  Gain1 : Gain  Gain=(Xd1 - Xd2)/(Xd1-Xls)^2
  Gain10 : Gain  Gain=Xq1 - Xls
  Gain11 : Gain  Gain=1/Tqo2
  Gain2 : Gain  Gain=Xd - Xd1
  Gain3 : Gain  Gain=1/Tdo1
  Gain4 : Gain  Gain=Xq1 - Xls
  Gain5 : Gain  Gain=(Xq1 - Xq2)/(Xq1 - Xls)^2
  Gain6 : Gain  Gain=Xq - Xq1
  Gain7 : Gain  Gain=1/Tqo1
  Gain8 : Gain  Gain=Xd1 - Xls
  Gain9 : Gain  Gain=1/Tdo2
  Integrator{,1..3} (4 alike) : Integrator
  Product{1..4} (4 alike) : Product
  Sum : Sum  Inputs=++-
  Sum1 : Sum  Inputs=+-
  Sum2 : Sum  Inputs=--+
  Sum3 : Sum  Inputs=+++
  Sum4 : Sum  Inputs=+-
  Sum5 : Sum  Inputs=-+
  Sum6 : Sum  Inputs=--+
  Sum7 : Sum  Inputs=---
  Eq1 : Outport
  Ed1 : Outport  Port=2
  Phi_1d : Outport  Port=3
  Phi_2q : Outport  Port=4
  wires:
  Product4/1 -> Integrator1/1
  Gain7/1 -> Product4/2
  [R_temp_delta] -> Product4/1
  Product2/1 -> Integrator/1
  Gain3/1 -> Product2/2
  [R_temp_delta] -> Product2/1
  Product1/1 -> Integrator3/1
  Gain11/1 -> Product1/2
  [R_temp_delta] -> Product1/1
  Product3/1 -> Integrator2/1
  Gain9/1 -> Product3/2
  [R_temp_delta] -> Product3/1
  Temp/1 -> [R_temp_delta]
  [Phi_1d] -> Sum/2
  Gain/1 -> Sum/1
  Integrator/1 -> Eq1/1, [Eq1]
  [Id] -> Gain/1
  [Eq1] -> Sum/3
  Sum/1 -> Gain1/1
  [Id] -> Sum1/1
  Gain1/1 -> Sum1/2
  Sum1/1 -> Gain2/1
  [Eq1] -> Sum2/1
  Gain2/1 -> Sum2/2
  [Efd] -> Sum2/3
  Sum2/1 -> Gain3/1
  Integrator1/1 -> Ed1/1, [Ed1]
  [Iq] -> Gain4/1
  Gain4/1 -> Sum3/1
  [Phi_2q] -> Sum3/2
  [Ed1] -> Sum3/3
  Sum3/1 -> Gain5/1
  [Iq] -> Sum4/1
  Gain5/1 -> Sum4/2
  Sum4/1 -> Gain6/1
  [Ed1] -> Sum5/1
  Gain6/1 -> Sum5/2
  Sum5/1 -> Gain7/1
  [Id] -> Gain8/1
  Gain8/1 -> Sum6/1
  [Phi_1d] -> Sum6/2
  [Eq1] -> Sum6/3
  Sum6/1 -> Gain9/1
  Integrator2/1 -> [Phi_1d], Phi_1d/1
  [Iq] -> Gain10/1
  Gain10/1 -> Sum7/1
  [Phi_2q] -> Sum7/2
  [Ed1] -> Sum7/3
  Sum7/1 -> Gain11/1
  Integrator3/1 -> [Phi_2q], Phi_2q/1
  Id/1 -> [Id]
  Iq/1 -> [Iq]
  Efd/1 -> [Efd]

== system Electrical787/ELECTRICAL SYS /Generation Unit P.M.1/Generator/Electromagnetic Torque Output Power ==
  note: Torque from Field Winding
  note: Torque from Damper Windings
  Id : Inport
  Iq : Inport  Port=2
  Eq1 : Inport  Port=3
  Ed1 : Inport  Port=4
  Phi_1d : Inport  Port=5
  Phi_2q : Inport  Port=6
  Gain : Gain  Gain=(Xd2 - Xls)/(Xd1 - Xls)
  Gain1 : Gain  Gain=(Xq2 - Xls)/(Xq1 - Xls)
  Gain2 : Gain  Gain=(Xd1 - Xd2)/(Xd1-Xls)
  Gain3 : Gain  Gain=(Xq1 - Xq2)/(Xq1-Xls)
  Gain4 : Gain  Gain=(Xq2 - Xd2)
  Product{,1..4} (5 alike) : Product  RndMeth=Zero
  Sum : Sum
  Sum1 : Sum  Inputs=+-+
  Sum2 : Sum
  TE : Outport
  wires:
  Id/1 -> [Id]
  Eq1/1 -> [Eq1]
  Ed1/1 -> [Ed1]
  Phi_1d/1 -> [Phi_1d]
  Phi_2q/1 -> [Phi_2q]
  Iq/1 -> [Iq]
  [Eq1] -> Product/1
  [Iq] -> Product/2
  Product/1 -> Gain/1
  [Ed1] -> Product1/1
  [Id] -> Product1/2
  Product1/1 -> Gain1/1
  [Iq] -> Product2/1
  [Phi_1d] -> Product2/2
  Product2/1 -> Gain2/1
  [Id] -> Product3/1
  [Phi_2q] -> Product3/2
  Product3/1 -> Gain3/1
  [Id] -> Product4/1
  [Iq] -> Product4/2
  Product4/1 -> Gain4/1
  Gain3/1 -> Sum1/2
  Gain2/1 -> Sum1/1
  Gain4/1 -> Sum1/3
  Gain/1 -> Sum/1
  Gain1/1 -> Sum/2
  Sum/1 -> Sum2/1
  Sum1/1 -> Sum2/2
  Sum2/1 -> TE/1

== system Electrical787/ELECTRICAL SYS /Generation Unit P.M.1/Generator/Generator Power Loss ==
  Ed : Inport
  Eq : Inport  Port=2
  Id : Inport  Port=3
  Iq : Inport  Port=4
  Te : Inport  Port=5
  w/ws : Inport  Port=6
  Bus Creator : BusCreator  Inputs=6
  Gain1 : Gain  Gain=SB
  Gain2 : Gain  Gain=SB
  Gain3 : Gain  Gain=SB
  Product : Product  RndMeth=Zero
  Product1 : Product  RndMeth=Zero
  Product2 : Product  RndMeth=Zero
  Sum1 : Sum  Inputs=-+
  Sum2 : Sum
  PE : Outport
  PM : Outport  Port=2
  PLOSS : Outport  Port=3
  m : Outport  Port=4
  wires:
  Ed/1 -> [Ed]
  Eq/1 -> [Eq]
  Id/1 -> [Id]
  Iq/1 -> [Iq]
  Te/1 -> [Te]
  w/ws/1 -> [nu]
  [Ed] -> Product/1
  [Id] -> Product/2
  [Eq] -> Product1/1
  [Iq] -> Product1/2
  [Te] -> Product2/1
  [nu] -> Product2/2
  Product/1 -> Sum2/1
  Product1/1 -> Sum2/2
  Sum2/1 -> Sum1/1, Gain1/1
  Product2/1 -> Sum1/2, Gain3/1
  Sum1/1 -> Gain2/1
  [Ed] -> Bus Creator/1  "Vd"
  [Id] -> Bus Creator/2  "Id"
  [Eq] -> Bus Creator/3  "Vq"
  [Iq] -> Bus Creator/4  "Iq"
  [Te] -> Bus Creator/5  "Te"
  [nu] -> Bus Creator/6  "nu"
  Bus Creator/1 -> m/1
  Gain2/1 -> PLOSS/1
  Gain1/1 -> PE/1
  Gain3/1 -> PM/1

== system Electrical787/ELECTRICAL SYS /Generation Unit P.M.1/Generator/Stator Voltage ==
  Id : Inport
  Iq : Inport  Port=2
  Eq1 : Inport  Port=3
  Ed1 : Inport  Port=4
  Phi_1d : Inport  Port=5
  Phi_2q : Inport  Port=6
  w/ws : Inport  Port=7
  Temp : Inport  Port=8
  Gain : Gain  Gain=(Xq2 - Xls)/(Xq1 - Xls)
  Gain1 : Gain  Gain=(Xq1 - Xq2)/(Xq1 - Xls)
  Gain2 : Gain  Gain=(Xq2 - Xd2)
  Gain3 : Gain  Gain=(Xd2 - Xls)/(Xd1 - Xls)
  Gain4 : Gain  Gain=(Xd1 - Xd2)/(Xd1 - Xls)
  Gain5 : Gain  Gain=Rs
  Gain6 : Gain  Gain=Xd2
  Gain7 : Gain  Gain=Rs
  Gain8 : Gain  Gain=Xd2
  Product{,1..3,5} (5 alike) : Product  RndMeth=Zero
  Product4 : Product
  Sum : Sum
  Sum1 : Sum  Inputs=+-+
  Sum2 : Sum  Inputs=--+
  Sum3 : Sum  Inputs=-++
  Ed : Outport
  Eq : Outport  Port=2
  wires:
  Iq/1 -> Gain6/1, Product5/2, Gain2/1
  Product5/1 -> Gain7/1
  Product4/1 -> Sum3/1
  Gain5/1 -> Product4/1
  Temp/1 -> Product4/2, Product5/1
  Gain2/1 -> Sum1/3
  Ed1/1 -> Gain/1
  Phi_2q/1 -> Gain1/1
  Eq1/1 -> Gain3/1
  Phi_1d/1 -> Gain4/1
  Gain4/1 -> Sum/2
  Gain3/1 -> Sum/1
  Gain/1 -> Sum1/1
  Gain1/1 -> Sum1/2
  Sum/1 -> Product/1
  Sum1/1 -> Product1/1
  w/ws/1 -> Product1/2, Product/2, Product3/2, Product2/1
  Product/1 -> Sum2/3
  Id/1 -> Gain5/1, Gain8/1
  Gain6/1 -> Product2/2
  Gain8/1 -> Product3/1
  Product1/1 -> Sum3/2
  Product2/1 -> Sum3/3
  Sum3/1 -> Ed/1  "Vd"
  Sum2/1 -> Eq/1  "Vq"
  Product3/1 -> Sum2/1
  Gain7/1 -> Sum2/2
